simulink model "projet"  (R2023a)
settings: Solver=VariableStepAuto  StartTime=0.0  StopTime=100  RelTol=1e-3
values from neighbouring files (symbols this model uses):
  a = 0.102    [initiation.m]
  b = 0    [initiation.m]
  c = 0.5    [initiation.m]
  d = 1    [initiation.m]
  f = 0.1    [initiation.m]
  K_delta = -1    [initiation.m]
  Kp = 5    [initiation.m]
  rayon = 2    [initiation.m]
  theta0 = 0    [initiation.m]
  x0 = 1    [initiation.m]
  y0 = 1.5    [initiation.m]
settings Model: Creator=Lelhadi2022  LastModifiedBy=lelhadi2022

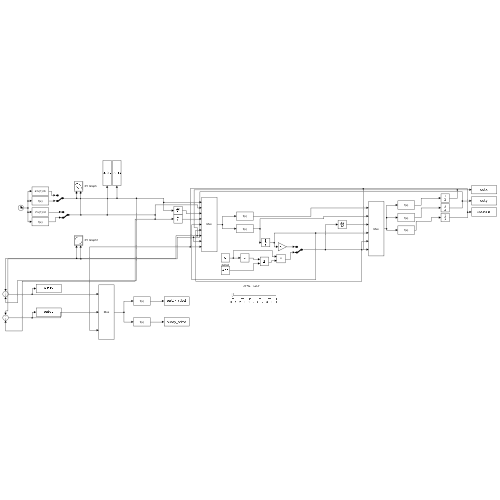
[thumbnail: Simulink's stored preview of the top-level diagram]
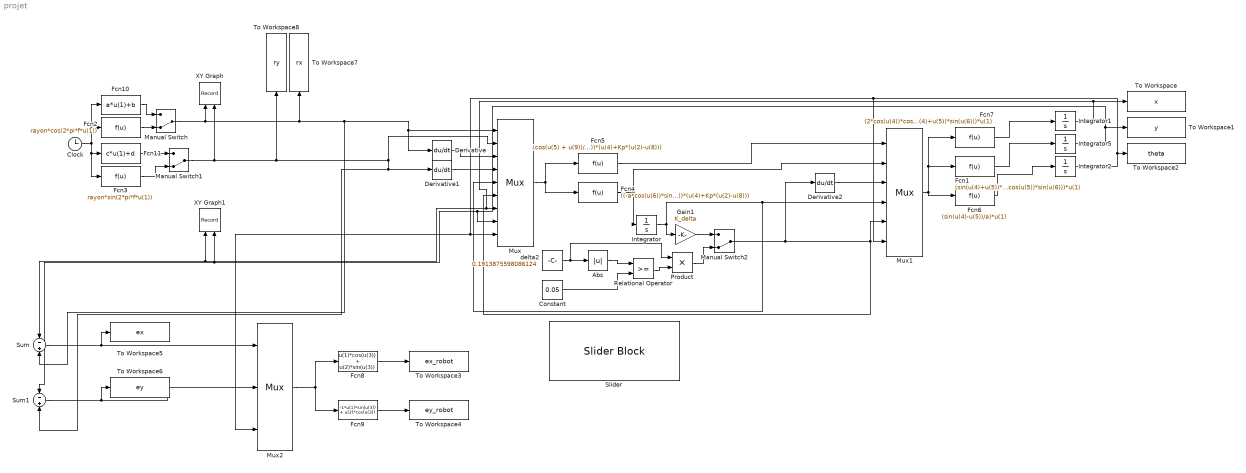
== system projet ==
  Abs : Abs  SaturateOnIntegerOverflow=off
  Clock : Clock
  Constant : Constant  Value=0.05
  Derivative : Derivative
  Derivative1 : Derivative
  Derivative2 : Derivative
  Fcn1 : Fcn  Expr=(sin(u(4)+u(5))*cos(u(6))+2*cos(u(4))*cos(u(5))*sin(u(6)))*u(1)
  Fcn10 : Fcn  Expr=a*u(1)+b
  Fcn11 : Fcn  Expr=c*u(1)+d
  Fcn2 : Fcn  Expr=rayon*cos(2*pi*f*u(1))
  Fcn3 : Fcn  Expr=rayon*sin(2*pi*f*u(1))
  Fcn4 : Fcn  Expr=((-a*cos(u(6))*sin(u(5)+u(9))-e*sin(u(5)-u(6))*cos(u(5)+u(9)))/(a*e*sin(u(5) + u(9))^2*cos(u(6)) + a*e*cos(u(6))*cos(u(5)+u(9))^2))*(u(3)+Kp*(u(1)-u(7)))+((a*cos(u(6))*cos(u(5)+u(9))-e*sin(u(5)-u(6))*sin(u(5)+u(9)))/(a*e*sin(u(5) + u(9))^2*cos(u(6)) + a*e*cos(u(6))*cos(u(5)+u(9))^2))*(u(4)+Kp*(u(2)-u(8)))
  Fcn5 : Fcn  Expr=(cos(u(5) + u(9))/(2*sin(u(5) + u(9))^2*cos(u(6)) + 2*cos(u(6))*cos(u(5) + u(9))^2))*(u(3)+Kp*(u(1)-u(7)))+(sin(u(5) +u(9))/(2*sin(u(5) + u(9))^2*cos(u(6))+2*cos(u(6))*cos(u(5)+u(9))^2))*(u(4)+Kp*(u(2)-u(8)))
  Fcn6 : Fcn  Expr=(sin(u(4)-u(5))/a)*u(1)
  Fcn7 : Fcn  Expr=(2*cos(u(4))*cos(u(5))*cos(u(6))-sin(u(4)+u(5))*sin(u(6)))*u(1)
  Fcn8 : Fcn  Expr=u(1)*cos(u(3)) + u(2)*sin(u(3))
  Fcn9 : Fcn  Expr=-1*u(1)*sin(u(3)) + u(2)*cos(u(3))
  Gain1 : Gain  Gain=K_delta
  Integrator : Integrator
  Integrator1 : Integrator  InitialCondition=x0
  Integrator2 : Integrator  InitialCondition=theta0
  Integrator5 : Integrator  InitialCondition=y0
  Manual Switch : ManualSwitch  CurrentSetting=0
  Manual Switch1 : ManualSwitch  CurrentSetting=0
  Manual Switch2 : ManualSwitch  CurrentSetting=0
  Mux : Mux  Inputs=9
  Mux1 : Mux  Inputs=6
  Mux2 : Mux  Inputs=3
  Product : Product
  Relational Operator : RelationalOperator  OutDataTypeStr=boolean  RndMeth=Simplest  InputSameDT=off
  Slider : SliderBlock  ScaleMax=10
  Sum : Sum  Inputs=-|+
  Sum1 : Sum  Inputs=-|+
  To Workspace : ToWorkspace  VariableName=x  SaveFormat=Timeseries  SampleTime=-1
  To Workspace1 : ToWorkspace  VariableName=y  SaveFormat=Timeseries  SampleTime=-1
  To Workspace2 : ToWorkspace  VariableName=theta  SaveFormat=Timeseries  SampleTime=-1
  To Workspace3 : ToWorkspace  VariableName=ex_robot  SaveFormat=Timeseries  SampleTime=-1
  To Workspace4 : ToWorkspace  VariableName=ey_robot  SaveFormat=Timeseries  SampleTime=-1
  To Workspace5 : ToWorkspace  VariableName=ex  SaveFormat=Timeseries  SampleTime=-1
  To Workspace6 : ToWorkspace  VariableName=ey  SaveFormat=Timeseries  SampleTime=-1
  To Workspace7 : ToWorkspace  VariableName=rx  SaveFormat=Timeseries  SampleTime=-1
  To Workspace8 : ToWorkspace  VariableName=ry  SaveFormat=Timeseries  SampleTime=-1
  XY Graph : Record  FileSettingsInternal="{\"entries\":[{\"content\":{\"excelSettings\":{\"content\":{},\"type\":\"Streamout.ExcelSettings\"}},\"type\":\"Streamout.FileSettingStorage\",\"uuid\":\"\"}],\"packageUris\":[\"http:\\/\\/schema.mathworks.com\\/mf0\\/streamout_blocks\\/R2020a\"],\"version\":\"1.0\"}"  Layout=[1 1]  SignalsInternal="{\"entries\":[{\"content\":{\"signals\":[{\"content\":{\"blockPath\":[],\"dimensions\":[1],\"domain\":\"\",\"lineColor\":\"#a2142f\",\"plots\":[1],\"port\":1,\"sid\":[\"\"],\"signalID\":1583,\"signalName\":\"Manual Switch\"},\"type\":\"RecordBlkView.Signal\",\"uuid\":\"\"},{\"content\":{\"blockPath\":[],\"dimensions\":[1],\"domain\":\"\",\"lineColor\":\"#139fff\",\"plots\":[1],\"port\":2,\"sid\":[\"\"],\"signalID\":1587,\"signalName\":\"Manual Switch1\"},\"type\":\"RecordBlkView.Signal\",\"uuid\":\"\"}]},\"type\":\"RecordBlkView.InputSignals\",\"uuid\":\"\"}],\"packageUris\":[\"http:\\/\\/schema.mathworks.com\\/mf0\\/streamout_blocks\\/R2020a\"],\"version\":\"1.0\"}"  VisualizationBindings="{\"xyplotplugin\":{\"info\":[{\"series\":[{\"bindingParametersList\":[{\"parameter\":\"X-Axis\",\"signalID\":1583,\"signalName\":\"Manual Switch\"},{\"parameter\":\"Y-Axis\",\"signalID\":1587,\"signalName\":\"Manual Switch1\"}],\"seriesID\":6684}],\"subplotID\":1}]}}"  CompatibilityTag=XY
  XY Graph1 : Record  FileSettingsInternal="{\"entries\":[{\"content\":{\"excelSettings\":{\"content\":{},\"type\":\"Streamout.ExcelSettings\"}},\"type\":\"Streamout.FileSettingStorage\",\"uuid\":\"\"}],\"packageUris\":[\"http:\\/\\/schema.mathworks.com\\/mf0\\/streamout_blocks\\/R2020a\"],\"version\":\"1.0\"}"  Layout=[1 1]  SignalsInternal="{\"entries\":[{\"content\":{\"signals\":[{\"content\":{\"blockPath\":[],\"dimensions\":[1],\"domain\":\"\",\"lineColor\":\"#a2142f\",\"plots\":[1],\"port\":1,\"sid\":[\"\"],\"signalID\":1591,\"signalName\":\"Integrator1\"},\"type\":\"RecordBlkView.Signal\",\"uuid\":\"\"},{\"content\":{\"blockPath\":[],\"dimensions\":[1],\"domain\":\"\",\"lineColor\":\"#139fff\",\"plots\":[1],\"port\":2,\"sid\":[\"\"],\"signalID\":1595,\"signalName\":\"Integrator5\"},\"type\":\"RecordBlkView.Signal\",\"uuid\":\"\"}]},\"type\":\"RecordBlkView.InputSignals\",\"uuid\":\"\"}],\"packageUris\":[\"http:\\/\\/schema.mathworks.com\\/mf0\\/streamout_blocks\\/R2020a\"],\"version\":\"1.0\"}"  VisualizationBindings="{\"xyplotplugin\":{\"info\":[{\"series\":[{\"bindingParametersList\":[{\"parameter\":\"X-Axis\",\"signalID\":1591,\"signalName\":\"Integrator1\"},{\"parameter\":\"Y-Axis\",\"signalID\":1595,\"signalName\":\"Integrator5\"}],\"seriesID\":16038}],\"subplotID\":1}]}}"  CompatibilityTag=XY
  delta2 : Constant  Value=0.1913875598086124
  wires:
  Mux/1 -> Fcn5/1, Fcn4/1
  Fcn5/1 -> Mux1/1
  Mux1/1 -> Fcn7/1, Fcn1/1, Fcn6/1
  Fcn7/1 -> Integrator1/1
  Fcn1/1 -> Integrator5/1
  Fcn6/1 -> Integrator2/1
  Manual Switch2/1 -> Derivative2/1, Mux/6, Mux1/5
  Integrator1/1 -> To Workspace/1, Sum/1, XY Graph1/1, Mux/7
  Integrator5/1 -> Mux/8, Sum1/1, XY Graph1/2, To Workspace1/1
  Integrator2/1 -> To Workspace2/1, Mux/9, Mux2/3, Mux1/6
  Fcn4/1 -> Mux1/2, Integrator/1
  Derivative1/1 -> Mux/4
  Derivative/1 -> Mux/3
  Clock/1 -> Fcn11/1, Fcn3/1, Fcn10/1, Fcn2/1
  Manual Switch/1 -> Derivative/1, Mux/1, Sum/2, To Workspace7/1, XY Graph/1
  Manual Switch1/1 -> Mux/2, Derivative1/1, Sum1/2, To Workspace8/1, XY Graph/2
  Sum/1 -> To Workspace5/1, Mux2/1
  Sum1/1 -> To Workspace6/1, Mux2/2
  Mux2/1 -> Fcn9/1, Fcn8/1
  Fcn8/1 -> To Workspace3/1
  Fcn9/1 -> To Workspace4/1
  Fcn2/1 -> Manual Switch/2
  Fcn3/1 -> Manual Switch1/2
  Fcn10/1 -> Manual Switch/1
  Fcn11/1 -> Manual Switch1/1
  Integrator/1 -> Mux/5, Mux1/4, Gain1/1
  Gain1/1 -> Manual Switch2/1
  Derivative2/1 -> Mux1/3
  delta2/1 -> Product/1, Abs/1
  Abs/1 -> Relational Operator/1
  Constant/1 -> Relational Operator/2
  Relational Operator/1 -> Product/2
  Product/1 -> Manual Switch2/2
